simulink model "Nieliniowy"  (R2015a)
settings: Solver=ode45  StartTime=0.0  StopTime=200  RelTol=1e-3  AbsTol=1e-6
values from neighbouring files (symbols this model uses):
  A1 = 3500    [Dodatkowe.m]    (also in Dodatkowe2.m; ZbiorniczkiLiniowe.m; ZbiorniczkiSumaryczne.m)
  A2 = 2000    [Dodatkowe.m]    (also in Dodatkowe2.m; ZbiorniczkiLiniowe.m; ZbiorniczkiSumaryczne.m)
  Aw1 = 0.1 * A1    (= 350)    [Dodatkowe.m]    (also in Dodatkowe2.m; ZbiorniczkiLiniowe.m; ZbiorniczkiSumaryczne.m)
  Aw2 = 0.1 * A2    (= 200)    [Dodatkowe.m]    (also in Dodatkowe2.m; ZbiorniczkiLiniowe.m; ZbiorniczkiSumaryczne.m)
  df1 = 200    [Dodatkowe.m]    (also in Dodatkowe2.m; ZbiorniczkiLiniowe.m; ZbiorniczkiSumaryczne.m)
  df2 = 0    [Dodatkowe.m]    (also in Dodatkowe2.m; ZbiorniczkiLiniowe.m; ZbiorniczkiSumaryczne.m)
  f1 = wektorf1(i)    [Dodatkowe.m]    (also in Dodatkowe2.m; ZbiorniczkiLiniowe.m; ZbiorniczkiSumaryczne.m)
  f2 = 0    [Dodatkowe.m]    (also in Dodatkowe2.m = 400; ZbiorniczkiLiniowe.m; ZbiorniczkiSumaryczne.m)
  g = 10    [Dodatkowe.m]    (also in Dodatkowe2.m; ZbiorniczkiLiniowe.m; ZbiorniczkiSumaryczne.m)
  h1 = ((f1.^2)/((Aw1.^2)*2*g))+((f1+f2).^2)/((Aw2.^2)*2*g)    [Dodatkowe.m]    (also in Dodatkowe2.m; ZbiorniczkiLiniowe.m = (f1/a1)+(f1+df2)/a2; ZbiorniczkiSumaryczne.m = (f1/a1)+(f1+df2)/a2)
  h2 = ((f1+f2).^2)/((Aw2.^2)*2*g)    [Dodatkowe.m]    (also in Dodatkowe2.m; ZbiorniczkiLiniowe.m = (f1+df2)/a2; ZbiorniczkiSumaryczne.m = (f1+df2)/a2)
  t1 = 40    [Dodatkowe.m]    (also in Dodatkowe2.m; ZbiorniczkiLiniowe.m; ZbiorniczkiSumaryczne.m)
  t2 = 40    [Dodatkowe.m]    (also in Dodatkowe2.m; ZbiorniczkiLiniowe.m; ZbiorniczkiSumaryczne.m)
settings Model: Creator=LAB320-1552  LastModifiedBy=apuch
settings DebuggingCC: UnderspecifiedInitializationDetection=Classic  MergeDetectMultiDrivingBlocksExec=none  StateNameClashWarn=warning  StrictBusMsg=ErrorOnBusTreatedAsVector

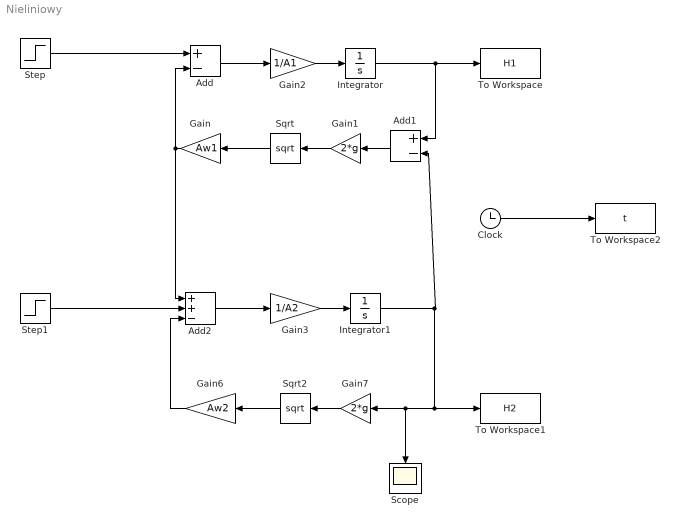
== system Nieliniowy ==
  Add : Sum  Inputs=+-
  Add1 : Sum  Inputs=+-
  Add2 : Sum  Inputs=++-
  Clock : Clock
  Gain : Gain  Gain=Aw1
  Gain1 : Gain  Gain=2*g
  Gain2 : Gain  Gain=1/A1
  Gain3 : Gain  Gain=1/A2
  Gain6 : Gain  Gain=Aw2
  Gain7 : Gain  Gain=2*g
  Integrator : Integrator  InitialCondition=h1
  Integrator1 : Integrator  InitialCondition=h2
  Scope : Scope
  Sqrt : Sqrt  SaturateOnIntegerOverflow=on
  Sqrt2 : Sqrt  SaturateOnIntegerOverflow=on
  Step : Step  Time=t1  Before=f1  After=f1+df1  SampleTime=0
  Step1 : Step  Time=t2  Before=f2  After=f2+df2  SampleTime=0
  To Workspace : ToWorkspace  VariableName=H1  SampleTime=-1
  To Workspace1 : ToWorkspace  VariableName=H2  SampleTime=-1
  To Workspace2 : ToWorkspace  VariableName=t  SampleTime=-1
  wires:
  Step/1 -> Add/1
  Add/1 -> Gain2/1
  Gain2/1 -> Integrator/1
  Gain1/1 -> Sqrt/1
  Sqrt/1 -> Gain/1
  Gain/1 -> Add/2, Add2/1
  Integrator/1 -> Add1/1, To Workspace/1
  Add1/1 -> Gain1/1
  Step1/1 -> Add2/2
  Add2/1 -> Gain3/1
  Gain3/1 -> Integrator1/1
  Integrator1/1 -> Scope/1, Gain7/1, To Workspace1/1, Add1/2
  Gain7/1 -> Sqrt2/1
  Sqrt2/1 -> Gain6/1
  Gain6/1 -> Add2/3
  Clock/1 -> To Workspace2/1
